simulink model "InvertedPendulum"  (R2024b)
settings: Solver=VariableStepAuto  StartTime=0.0  StopTime=10.0  RelTol=1e-3
model workspace (MAT data in the model file):
  C = [1  0  0  0; 0  0  1  0]
  D = [0; 0]
  I = 0.006
  M = 0.5
  b = 0.1
  g = 9.8
  l = 0.3
  m = 0.2
undefined symbols (not defined in the file): A, B, Continuous, Time
libraries: simulink x2, ctrlSharedLib x1
settings Model: Creator=shukl  LastModifiedBy=shukl

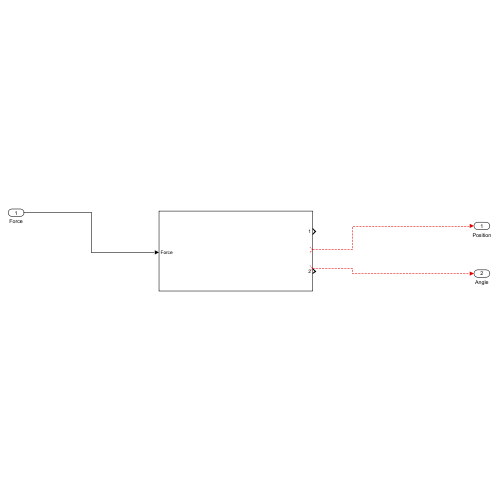
[thumbnail: Simulink's stored preview of the top-level diagram]
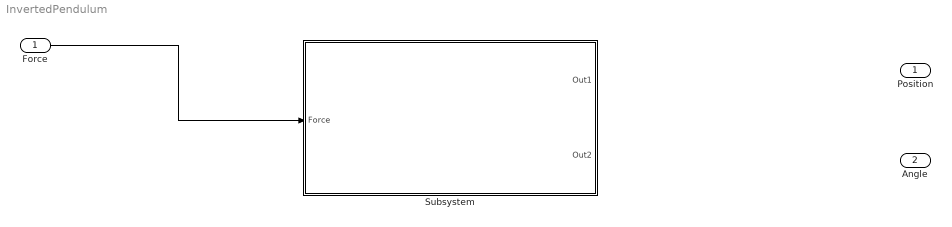
== system InvertedPendulum ==
  Force : Inport
  Subsystem : Subsystem  LoadFcn=|  InitFcn=|
      LoadFcn=|
      | M = 0.5;
      | m = 0.2;
      | l = 0.3;
      | I = 0.006;
      | b = 0.1;
      | g = 9.8;
      | 
      | p = I*(M + m) + M*m*l^2;
      | 
      | A = [ 0 1 0 0;
      |       0 -((I + m*l^2)*b)/p (m^2 * g * l^2)/p 0;
      |       0 0 0 1;
      |       0 -(m * l * b)/p m * g * l * (M + m)/p 0 ];
      | 
      | B = [ 0;
      |       (I + m * l^2)/p;
      |       0;
      |       (m * l)/p ];
      | 
      | C = [1 0 0 0;
      |      0 0 1 0];
      | 
      | D = [0; 0];
      InitFcn=|
      | % Load physical parameters
      | M = 0.5;
      | m = 0.2;
      | l = 0.3;
      | I = 0.006;
      | b = 0.1;
      | g = 9.8;
      | 
      | % Composite moment
      | p = I*(M + m) + M*m*l^2;
      | 
      | % State-space matrices
      | A = [0 1 0 0;
      |      0 -((I + m*l^2)*b)/p (m^2 * g * l^2)/p 0;
      |      0 0 0 1;
      |      0 -(m * l * b)/p m * g * l * (M + m)/p 0];
      | 
      | B = [0;
      |      (I + m * l^2)/p;
      |      0;
      |      m * l / p];
      | 
      | C = [1 0 0 0;
      |      0 0 1 0];
      | 
      | D = [0;
      |      0];
  Position : Outport
  Angle : Outport  Port=2
  wires:
  Force/1 -> Subsystem/1(Force)
  ? -> Position/1
  ? -> Angle/1

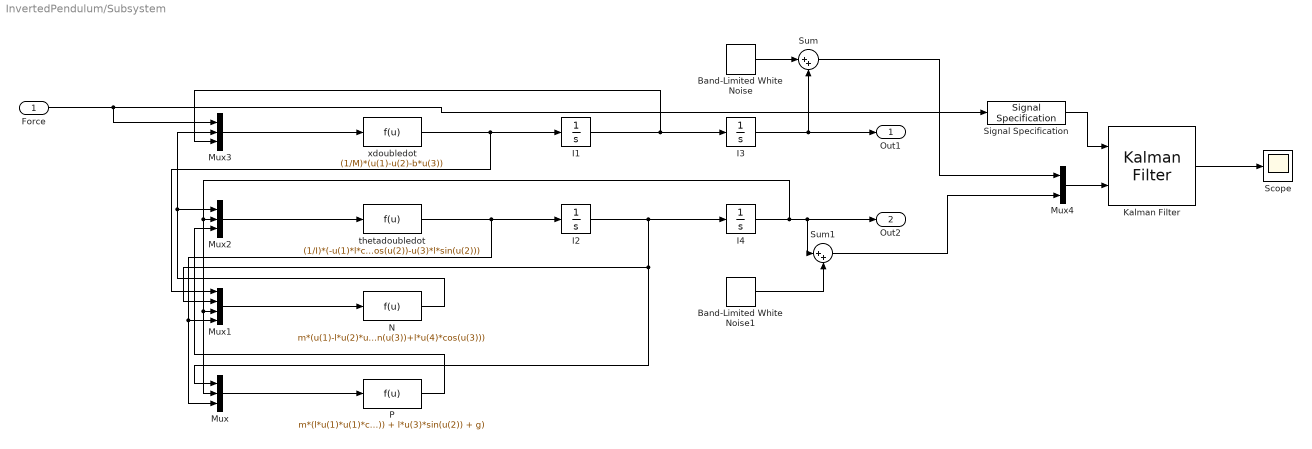
== system InvertedPendulum/Subsystem ==
  Force : Inport
  Band-Limited White Noise : simulink/Sources/Band-Limited White Noise  Cov=[0.1]  Ts=0.1  seed=[23341]
  Band-Limited White Noise1 : simulink/Sources/Band-Limited White Noise  Cov=[0.1]  Ts=0.1  seed=[23341]
  I1 : Integrator
  I2 : Integrator  InitialCondition=pi
  I3 : Integrator
  I4 : Integrator  InitialCondition=pi
  Kalman Filter : ctrlSharedLib/Kalman Filter  TimeDomain=Continuous-Time  UseCurrentEstimator=on  ModelSource=Individual A, B, C, D matrices  ModelSourceVariable=ss(0.95,1,1,0,1)  A=A  B=B  C=C  D=D  NumberOfStates=4  NumberOfInputs=1  NumberOfOutputs=2  InitialEstimateSource=Dialog  X0=[0; 0; 0; 0]  P0=10  UseK=off  UseGH=off  NumberOfProcessNoiseInputs=1  G=1  TimeInvariantG=on  H=0  TimeInvariantH=on  Q=1e-5 * eye(4)  TimeInvariantQ=on  R=1e-2 * eye(2)  TimeInvariantR=on  N=0  TimeInvariantN=on  AddInputPort=on  AddEnablePort=off  OutputEstimatedY=off  OutputP=off  Ts=0.01
  Mux : Mux  Inputs=3
  Mux1 : Mux
  Mux2 : Mux  Inputs=3
  Mux3 : Mux  Inputs=3
  Mux4 : Mux  Inputs=2
  N : Fcn  Expr=m*(u(1)-l*u(2)*u(2)*sin(u(3))+l*u(4)*cos(u(3)))
  P : Fcn  Expr=m*(l*u(1)*u(1)*cos(u(2)) + l*u(3)*sin(u(2)) + g)
  Scope : Scope
  Signal Specification : SignalSpecification  Dimensions=1
  Sum : Sum  Inputs=|++
  Sum1 : Sum  Inputs=|++
  thetadoubledot : Fcn  Expr=(1/I)*(-u(1)*l*cos(u(2))-u(3)*l*sin(u(2)))
  xdoubledot : Fcn  Expr=(1/M)*(u(1)-u(2)-b*u(3))
  Out1 : Outport
  Out2 : Outport  Port=2
  wires:
  Mux3/1 -> xdoubledot/1
  thetadoubledot/1 -> Mux/3, Mux1/4, I2/1
  xdoubledot/1 -> Mux1/1, I1/1
  I4/1 -> Out2/1, Sum1/1, Mux/2, Mux1/3, Mux2/2
  N/1 -> Mux3/2, Mux2/1
  P/1 -> Mux2/3
  I1/1 -> Mux3/3, I3/1
  I2/1 -> Mux/1, Mux1/2, I4/1
  Mux2/1 -> thetadoubledot/1
  Mux1/1 -> N/1
  Mux/1 -> P/1
  I3/1 -> Out1/1, Sum/2
  Mux4/1 -> Kalman Filter/2
  Band-Limited White Noise/1 -> Sum/1
  Band-Limited White Noise1/1 -> Sum1/2
  Sum/1 -> Mux4/1
  Sum1/1 -> Mux4/2
  Kalman Filter/1 -> Scope/1
  Force/1 -> Signal Specification/1, Mux3/1
  Signal Specification/1 -> Kalman Filter/1
